simulink model "slvnvdemo_fuelsys_doorsreq"  (Simulink 7.6)
settings: Solver=ode45  SolverMode=SingleTasking  StartTime=0.0  StopTime=20  FixedStep=0.001  RelTol=1e-5  AbsTol=1e-6
model workspace (MAT data in the model file):
  A1 = [1 -0.740818220682]
  A2 = [1 -0.740818220682]
  A3 = [1 0 0 0]
  B1 = [8.76963147833 -8.51044969901]
  B2 = [0 0.259181779318]
  B3 = [1 0 0 0]
  DISABLED = 3
  hys = 25
  Ki = 0.012
  LOW = 1
  max_ego = 1.2
  max_press = 1
  max_speed = 628
  max_throt = 90
  min_press = 0.001
  min_throt = 3
  o2_t_thresh = 4.8
  press = [0.05 0.1 0.15 0.2 0.25 0.3 0.35 0.4 0.45 0.5 0.55 0.6 0.65 0.7 0.75 0.8 0.85 0.9 0.95]
  PressEst = [0.806253176324 0.553142316929 0.37151500209 0.277667903103 0.220198954207 0.181288665766 0.153200000489 0.115431020872 0.0913067476324 0.0746519188607 0.0625231108324 0.0533383634277 ... (306 elements, 18x17)]
  pumpCon = [-0.0556348 -0.0022828 0.0256932 0.0435188 0.0562692 0.0661194857143 0.0741572 0.08697 0.0972452 0.106070342857 0.1139892 0.121303866667 ... (342 elements, 18x19)]
  RICH = 2
  SpeedEst = [471.837839721 550.80940091 777.559313277 1080.9243499 1418.36795322 1769.7468768 2125.37309264 2480.20345067 2831.37796793 3177.14006959 3516.32917143 4064.90417867 ... (323 elements, 17x19)]
  SpeedVect = [50 75 100 125 150 175 200 250 300 350 400 450 500 600 700 800 900 1000]
  ThrotEst = [0 0 0 0 0 0 0 0 0 0 0 0 ... (342 elements, 18x19)]
  ThrotVect = [0 3 6 9 12 15 18 21 24 27 30 35 46 57 68 79 90]
  xzero = [0.0684931506849; 0.1; 0; 0]
  zero_thresh : num (value not decoded)
undefined symbols (not defined in the file or in its folder): DiscIntNeverNeededParam, sigbuilder_block
libraries: simulink x4, simulink_extras x3
Description:
  | This is a model of a fuel control system where Stateflow(R) is used to handle the fault management of the system.  The system modeled here contains four separate sensors: a throttle sensor, a speed sensor, an oxygen sensor, and a pressure sensor.  Each of these sensors is represented by a parallel state in Stateflow.  Each parallel state contains two substates, a normal state and a failed state (the exception being the oxygen sensor, which also contains a warmup state).
  | 
  | If any of the sensor readings is outside an acceptable range, then a fault is registered in Stateflow, and the substate of the corresponding subsystem transitions to the failed state.  If a subsystem recovers, it can transition back to the normal state.  The number of failures in the system at any given time is represented in the Sens_Failure_Counter parallel state.
  | 
  | The last parallel state in the Stateflow chart is called Fueling_Mode.  This state regulates the oxygen to fuel mixture ratio.  If a failure is detected, then the oxygen to fuel ratio is increased.  If multiple failures are detected, then the fuel system is disabled until there are no longer multiple failures in the system.
settings Model: RequirementInfo={'doors' '00001143' '1' 'false' 'DOORS Surrogate Item' '' ; 'other' 'fuelsys_req_docs\slvnvdemo_FuelSys_DesignDescription.docx' '' 'true' 'Design Description Microsoft Word Document' '' } %GIDa_b9f5e970_9947_4c5b_8209_982c9caa298e  reqMgrSettings="100 S'doors','misc'{{S'surrogatepath','savemodel','savesurrogate','updateLinks','doorsLinks2sl','slLinks2Doors','purgeDoors','purgeSimulink','detaillevel','surrogateId','synctime'{{T\"/DemoRMI/slvnvdemo_fuelsys_doorsreq\",M[0],M[0],M[0],M[0],M[0],M[0],M[0],M[6],T\"00001143\",T\"\"}},S'mode','pathStorage'{{T\"generic\",T\"modelRelative\"}}}}"  Creator=The MathWorks Inc.  CovMetricSettings=dcmtr  ExtModeTrigMode=oneshot  ExtModeArmWhenConnect=off  ExtModeAutoUpdateStatusClock=off
settings SolverCC: InsertRTBMode=Auto
settings DataIOCC: LimitDataPoints=off  SaveOutput=off  SaveTime=off
settings OptimizationCC: InlineInvariantSignals=on  InitFltsAndDblsToZero=on  EfficientMapNaN2IntZero=off
settings DebuggingCC: SaveWithParameterizedLinksMsg=none  SignalResolutionControl=TryResolveAllWithWarning  SolverPrmCheckMsg=none  MultiTaskDSMMsg=warning  MultiTaskCondExecSysMsg=none  IntegerOverflowMsg=none  StrictBusMsg=None
settings HardwareCC: TargetUnknown=on
settings SFSimCC: SimParseCustomCode=off
settings RTWCC: IncludeERTFirstTime=on
settings GRTTargetCC: TargetFcnLib=ansi_tfl_tmw.mat

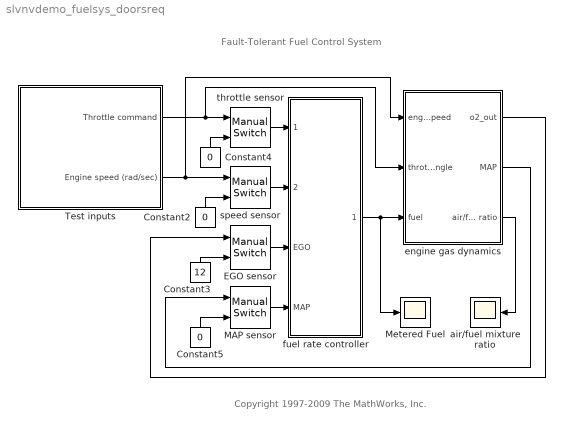
== system slvnvdemo_fuelsys_doorsreq ==
  note: Fault-Tolerant Fuel Control System
  note: Copyright 1997-2009 The MathWorks, Inc.
  Constant2 : Constant  RequirementInfo={'doors' '00001143' '2' 'false' 'DOORS Surrogate Item' '' } %GIDa_6f510076_839c_4984_a068_82184ea5f27a  Value=0
  Constant3 : Constant  RequirementInfo={'doors' '00001143' '3' 'false' 'DOORS Surrogate Item' '' } %GIDa_4aea0302_c695_4d64_8fee_9965b0b11529  Value=12
  Constant4 : Constant  RequirementInfo={'doors' '00001143' '4' 'false' 'DOORS Surrogate Item' '' } %GIDa_f16c33ef_29fe_45bd_a15f_c77a44a505fb  Value=0
  Constant5 : Constant  RequirementInfo={'doors' '00001143' '5' 'false' 'DOORS Surrogate Item' '' } %GIDa_53ad70e6_a414_4a38_8170_e2a41f36da5c  Value=0
  EGO sensor : simulink/Signal Routing/Manual Switch  RequirementInfo={'doors' '00001143' '6' 'false' 'DOORS Surrogate Item' '' } %GIDa_fc1de3a5_f710_44ee_8aab_8ba6d02ce341  SystemSampleTime=-1  sw=1  action=0  varsize=off
  MAP sensor : simulink/Signal Routing/Manual Switch  RequirementInfo={'doors' '00001143' '7' 'false' 'DOORS Surrogate Item' '' } %GIDa_9fc2c968_6068_49c6_968d_b08e363248b9  SystemSampleTime=-1  sw=1  action=0  varsize=off
  Metered Fuel : Scope
      settings: RequirementInfo={'doors' '00001143' '8' 'false' 'DOORS Surrogate Item' '' } %GIDa_681a171d_a3c5_4885_b64c_8848497df52d  TickLabels=on  TimeRange=20  YMin=0.75  YMax=2.25  DataFormat=Array
  Test inputs : Subsystem  Tag=STV Subsys  RequirementInfo={'doors' '00001143' '9' 'false' 'DOORS Surrogate Item' '' ; 'doors' '00001143' '10' 'false' 'DOORS Surrogate Item' '' } %GIDa_edea01b3_1c6d_4155_a72f_5a035e20164d  LoadFcn=sigbuilder_block('load');  StartFcn=sigbuilder_block('start');  StopFcn=sigbuilder_block('stop');  ClipboardFcn=sigbuilder_block('clipboard');  mask(Sigbuilder block){}
      mask help: Create and generate interchangeable groups of signals whose waveforms are piecewise linear.
      mask init:
      | if ~strcmp(get_param(bdroot(gcbh),'SimulationStatus'),'stopped') tuvar = sigbuilder_block('maskInit'); end
      settings: CopyFcn=sigbuilder_block('copy');  DeleteFcn=sigbuilder_block('delete');  ModelCloseFcn=sigbuilder_block('modelClose');  PreSaveFcn=sigbuilder_block('preSave');  NameChangeFcn=sigbuilder_block('namechange');  OpenFcn=sigbuilder_block('open',[764.25 127.5 550.5 399.75 ]);  CloseFcn=sigbuilder_block('close');
      mask Display: plot(0,0,100,100,[10,10,40,40,10],[80,20,20,80,80],[40,10],[50,50], [40,27,10],[65,72,56],[40,25,25,10],[28,28,43,43]);
  air/fuel mixture ratio : Scope
      settings: RequirementInfo={'doors' '00001143' '11' 'false' 'DOORS Surrogate Item' '' } %GIDa_eb27b04a_0dbf_4cdf_926f_da0d02353e65  TickLabels=on  TimeRange=20  YMin=11  YMax=16  DataFormat=Array
  engine gas dynamics : Subsystem  RequirementInfo={'doors' '00001143' '12' 'false' 'DOORS Surrogate Item' '' } %GIDa_1a392509_8e3f_4212_812a_096eaacb0e7b
  fuel rate controller : Subsystem  RequirementInfo={'doors' '00001143' '61' 'false' 'DOORS Surrogate Item' '' } %GIDa_1c1b78ad_f226_4b22_a092_d4af30d7278c
  speed sensor : simulink/Signal Routing/Manual Switch  RequirementInfo={'doors' '00001143' '234' 'false' 'DOORS Surrogate Item' '' } %GIDa_db4c3198_d72b_4db1_84d1_60b53fad8198  SystemSampleTime=-1  sw=1  action=0  varsize=off
  throttle sensor : simulink/Signal Routing/Manual Switch  RequirementInfo={'doors' '00001143' '235' 'false' 'DOORS Surrogate Item' '' } %GIDa_38ef20e4_d6ae_4cd9_b31a_0da7b200996a  SystemSampleTime=-1  sw=1  action=0  varsize=off
  wires:
  engine gas dynamics/3(air/fuel ratio) -> air/fuel mixture ratio/1
  Test inputs/2(Engine speed (rad/sec)) -> engine gas dynamics/1(engine speed), speed sensor/1
  MAP sensor/1 -> fuel rate controller/4(MAP)
  EGO sensor/1 -> fuel rate controller/3(EGO)
  speed sensor/1 -> fuel rate controller/2(engine speed)
  throttle sensor/1 -> fuel rate controller/1(throttle)
  fuel rate controller/1(fuel rate) -> engine gas dynamics/3(fuel), Metered Fuel/1
  engine gas dynamics/1(o2_out) -> EGO sensor/1
  Constant5/1 -> MAP sensor/2
  Constant3/1 -> EGO sensor/2
  Test inputs/1(Throttle command) -> engine gas dynamics/2(throttle angle), throttle sensor/1
  Constant2/1 -> speed sensor/2
  Constant4/1 -> throttle sensor/2
  engine gas dynamics/2(MAP) -> MAP sensor/1

== system slvnvdemo_fuelsys_doorsreq/Test inputs ==
  Demux : Demux  Tag=STV Demux  Outputs=2
  FromWs : FromWorkspace  Tag=STV FromWs  VariableName=tuvar  SampleTime=0  SigBuilderData=DataTag1  VnvData=DataTag2
      SigBuilderData=|
      | common.afterFinalStr = 'Extrapolate'
      | common.sampleTime = 0
      | dataSet(1).timeRange = [0 20]
      | dataSet(1).name = 'Normal operation'
      | dataSet(2).timeRange = [0 20]
      | dataSet(2).name = 'RPM sensor failure'
      | sbobj.Groups(1).Name = 'Normal operation'
      | sbobj.Groups(1).Signals(1).Name = 'Throttle command'
      | sbobj.Groups(1).Signals(1).XData = [0 0.5 1 1.5 2 2.5 3 3.5 4 4.5 5 5.5 6 6.5 7 7.5 8 8.5 9 9.5 10 10.5 11 11.5 12 12.5 13 13.5 14 14.5 15 15.5 16 16.5 17 17.5 18 18.5 19 19.5 20]
      | sbobj.Groups(1).Signals(1).YData = [15 18.5355339059 20 18.5355339059 15 11.4644660941 10 11.4644660941 15 18.5355339059 20 18.5355339059 15 11.4644660941 10 11.4644660941 15 18.5355339059 20 18.5355339059 15 11.4644660941 10 11.4644660941 15 18.5355339059 20 18.5355339059 15 11.4644660941 10 11.4644660941 15 18.5355339059 20 18.5355339059 15 11.4644660941 10 11.4644660941 15]
      | sbobj.Groups(1).Signals(2).Name = 'Engine speed (rad/sec)'
      | sbobj.Groups(1).Signals(2).XData = [0 20]
      | sbobj.Groups(1).Signals(2).YData = [300 300]
      | sbobj.Groups(2).Name = 'RPM sensor failure'
      | sbobj.Groups(2).Signals(1).Name = 'Throttle command'
      | sbobj.Groups(2).Signals(1).XData = [0 0.5 1 1.5 2 2.5 3 3.5 4 4.5 5 5.5 6 6.5 7 7.5 8 8.5 9 9.5 10 10.5 11 11.5 12 12.5 13 13.5 14 14.5 15 15.5 16 16.5 17 17.5 18 18.5 19 19.5 20]
      | sbobj.Groups(2).Signals(1).YData = [15 18.5355339059 20 18.5355339059 15 11.4644660941 10 11.4644660941 15 18.5355339059 20 18.5355339059 15 11.4644660941 10 11.4644660941 15 18.5355339059 20 18.5355339059 15 11.4644660941 10 11.4644660941 15 18.5355339059 20 18.5355339059 15 11.4644660941 10 11.4644660941 15 18.5355339059 20 18.5355339059 15 11.4644660941 10 11.4644660941 15]
      | sbobj.Groups(2).Signals(2).Name = 'Engine speed (rad/sec)'
      | sbobj.Groups(2).Signals(2).XData = [0 10 10 14 14 20]
      | sbobj.Groups(2).Signals(2).YData = [300 300 700 700 300 300]
  Throttle command : Outport  Tag=STV Outport
  Engine speed (rad/sec) : Outport  Tag=STV Outport  Port=2
  wires:
  Demux/1 -> Throttle command/1
  FromWs/1 -> Demux/1
  Demux/2 -> Engine speed (rad/sec)/1

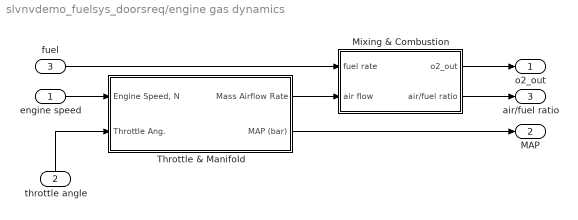
== system slvnvdemo_fuelsys_doorsreq/engine gas dynamics ==
  engine speed : Inport  RequirementInfo={'doors' '00001143' '13' 'false' 'DOORS Surrogate Item' '' } %GIDa_af43e267_eca7_4317_9a9e_118e96c8df3a
  throttle angle : Inport  RequirementInfo={'doors' '00001143' '14' 'false' 'DOORS Surrogate Item' '' } %GIDa_e17f4ea5_0288_401d_90f7_37f91cb17cef  Port=2
  fuel : Inport  RequirementInfo={'doors' '00001143' '15' 'false' 'DOORS Surrogate Item' '' } %GIDa_51f9453d_90e5_4716_8a70_66d58a29b78f  Port=3
  Mixing & Combustion : Subsystem  RequirementInfo={'doors' '00001143' '16' 'false' 'DOORS Surrogate Item' '' } %GIDa_b39f573e_5037_443c_be2b_1a4548c5c0e7
  Throttle & Manifold : Subsystem  RequirementInfo={'doors' '00001143' '26' 'false' 'DOORS Surrogate Item' '' } %GIDa_a2d66e4e_7a50_46f2_8e9d_462815b41651
  o2_out : Outport  RequirementInfo={'doors' '00001143' '58' 'false' 'DOORS Surrogate Item' '' } %GIDa_2b902bd2_437a_4448_b4ab_a1d7bbca09e4  InitialOutput=0
  MAP : Outport  RequirementInfo={'doors' '00001143' '59' 'false' 'DOORS Surrogate Item' '' } %GIDa_84abcf36_567c_4069_a0b2_4759d3edc095  Port=2  InitialOutput=0
  air/fuel ratio : Outport  RequirementInfo={'doors' '00001143' '60' 'false' 'DOORS Surrogate Item' '' } %GIDa_a523c5d4_fa31_4aa3_8903_8b83a3fe08ed  Port=3  InitialOutput=0
  wires:
  Throttle & Manifold/1(Mass Airflow Rate) -> Mixing & Combustion/2(air flow)
  fuel/1 -> Mixing & Combustion/1(fuel rate)
  engine speed/1 -> Throttle & Manifold/1("Engine Speed, N")
  throttle angle/1 -> Throttle & Manifold/2(Throttle Ang.)
  Mixing & Combustion/2(air/fuel ratio) -> air/fuel ratio/1
  Throttle & Manifold/2(MAP (bar)) -> MAP/1
  Mixing & Combustion/1(o2_out) -> o2_out/1

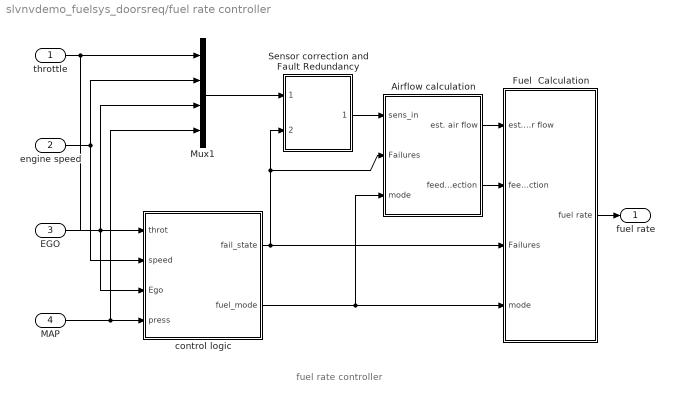
== system slvnvdemo_fuelsys_doorsreq/fuel rate controller ==
  note: fuel rate controller
  throttle : Inport  RequirementInfo="{'doors' '00001143' '62' 'false' 'DOORS Surrogate Item' '' ; 'linktype_rmi_doors' '00001140 (/DemoRMI/FuelSys Design Description)' '#24' 'true' '1.1.1.1  Throttle Sensor' 'design' } %GIDa_9cf99e51_43b0_47f7_8264_f2235da8c515"
  engine speed : Inport  RequirementInfo={'doors' '00001143' '63' 'false' 'DOORS Surrogate Item' '' } %GIDa_5b17eedf_e9cf_48a4_ac44_7982ccd64ca2  Port=2
  EGO : Inport  RequirementInfo={'doors' '00001143' '64' 'false' 'DOORS Surrogate Item' '' } %GIDa_6fef81ac_5f90_4a8e_828a_423a97d08b10  Port=3
  MAP : Inport  RequirementInfo="{'doors' '00001143' '65' 'false' 'DOORS Surrogate Item' '' ; 'linktype_rmi_doors' '00001140 (/DemoRMI/FuelSys Design Description)' '#28' 'true' '1.1.1.2  Manifold Absolute Pressure Sensor ' 'design' } %GIDa_4c5e0388_e181_4bd6_b11e_64e9ecd3fbd1"  Port=4
  Airflow calculation : Subsystem  RequirementInfo="{'doors' '00001143' '66' 'false' 'DOORS Surrogate Item' '' ; 'linktype_rmi_doors' '00001140 (/DemoRMI/FuelSys Design Description)' '#47' 'true' '1.2.1  Mass airflow estimation ' 'design' } %GIDa_e5d50a88_c804_4174_8af1_23d9a3e696a6"
  Fuel  Calculation : Subsystem  RequirementInfo={'doors' '00001143' '92' 'false' 'DOORS Surrogate Item' '' } %GIDa_34097df7_79d7_4c80_bbb4_c8c21d1d631f
  Mux1 : Mux  RequirementInfo={'doors' '00001143' '134' 'false' 'DOORS Surrogate Item' '' } %GIDa_83488a2d_fa56_4d28_96fb_fd2056fe6956
  Sensor correction and Fault Redundancy : Subsystem  RequirementInfo={'doors' '00001143' '135' 'false' 'DOORS Surrogate Item' '' } %GIDa_518d74c7_343f_4c0b_a3e5_2212a7618a1e
  control logic : Stateflow chart  Description=Stateflow diagram to determine control system operating mode  RequirementInfo={'doors' '00001143' '168' 'false' 'DOORS Surrogate Item' '' } %GIDa_5c71245a_39cc_4b2d_a7dc_93f0d532609e  TreatAsAtomicUnit=on
  fuel rate : Outport  RequirementInfo={'doors' '00001143' '233' 'false' 'DOORS Surrogate Item' '' } %GIDa_b9667016_fb09_447c_b6a0_1390dfc20aea  InitialOutput=0
  wires:
  MAP/1 -> Mux1/4, control logic/4(press)
  EGO/1 -> Mux1/3, control logic/3(Ego)
  engine speed/1 -> Mux1/2, control logic/2(speed)
  throttle/1 -> Mux1/1, control logic/1(throt)
  Mux1/1 -> Sensor correction and Fault Redundancy/1(Sensors)
  control logic/2(fuel_mode) -> Fuel  Calculation/4(mode), Airflow calculation/3(mode)
  Airflow calculation/2(feedback correction) -> Fuel  Calculation/2(feedback correction)
  Fuel  Calculation/1(fuel rate) -> fuel rate/1
  Airflow calculation/1(est. air flow) -> Fuel  Calculation/1(est. air flow)
  Sensor correction and Fault Redundancy/1(Corrected) -> Airflow calculation/1(sens_in)
  control logic/1(fail_state) -> Sensor correction and Fault Redundancy/2(Failures), Airflow calculation/2(Failures), Fuel  Calculation/3(Failures)

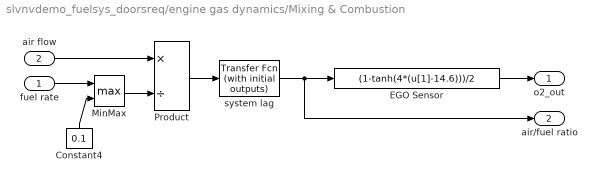
== system slvnvdemo_fuelsys_doorsreq/engine gas dynamics/Mixing & Combustion ==
  fuel rate : Inport  RequirementInfo={'doors' '00001143' '17' 'false' 'DOORS Surrogate Item' '' } %GIDa_a0da4f9a_920a_433c_bc96_8906b222f2c5
  air flow : Inport  RequirementInfo={'doors' '00001143' '18' 'false' 'DOORS Surrogate Item' '' } %GIDa_5caa34b4_a16f_4465_a750_f963464c11ad  Port=2
  Constant4 : Constant  RequirementInfo={'doors' '00001143' '19' 'false' 'DOORS Surrogate Item' '' } %GIDa_2bd17625_1ccb_44ba_a95c_a9230dfb67c2  Value=0.1
  EGO Sensor : Fcn  RequirementInfo={'doors' '00001143' '20' 'false' 'DOORS Surrogate Item' '' } %GIDa_6af401bd_9892_45e5_a1d1_0ec7c7cf995e  Expr=(1-tanh(4*(u[1]-14.6)))/2
  MinMax : MinMax  RequirementInfo={'doors' '00001143' '21' 'false' 'DOORS Surrogate Item' '' } %GIDa_6d9700e5_4410_4a4b_83fd_395721c529a2  Function=max  Inputs=2  SaturateOnIntegerOverflow=on  InputSameDT=on
  Product : Product  RequirementInfo={'doors' '00001143' '22' 'false' 'DOORS Surrogate Item' '' } %GIDa_088236aa_e2e4_4ea4_9127_1588bf7dce42  Inputs=*/  SaturateOnIntegerOverflow=on  RndMeth=Zero  InputSameDT=on  OutDataTypeStr=Inherit: Same as first input
  system lag : simulink_extras/Additional Linear/Transfer Fcn (with initial outputs)  RequirementInfo={'doors' '00001143' '23' 'false' 'DOORS Surrogate Item' '' } %GIDa_4fc8d989_be95_4469_a582_179e8d71f6fb  SystemSampleTime=-1  N=3  D=[1 3]  Y0=1/14.6  U0=1/14.6
  o2_out : Outport  RequirementInfo={'doors' '00001143' '24' 'false' 'DOORS Surrogate Item' '' } %GIDa_db90f587_e1ae_4b5c_a93b_c6026d9cd193  InitialOutput=0
  air/fuel ratio : Outport  RequirementInfo={'doors' '00001143' '25' 'false' 'DOORS Surrogate Item' '' } %GIDa_ccc3460d_06a5_47de_9c88_91db6cd6257a  Port=2  InitialOutput=0
  wires:
  Constant4/1 -> MinMax/2
  fuel rate/1 -> MinMax/1
  MinMax/1 -> Product/2
  Product/1 -> system lag/1
  system lag/1 -> air/fuel ratio/1, EGO Sensor/1
  EGO Sensor/1 -> o2_out/1
  air flow/1 -> Product/1

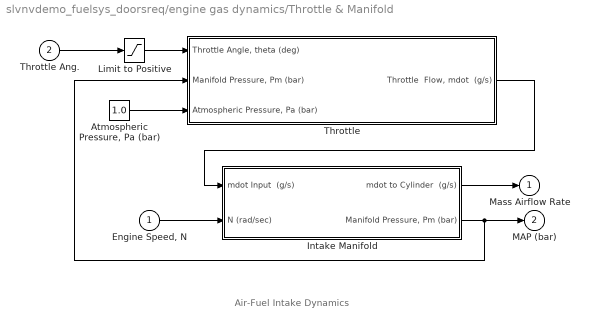
== system slvnvdemo_fuelsys_doorsreq/engine gas dynamics/Throttle & Manifold ==
  note: Air-Fuel Intake Dynamics
  "Engine Speed, N" : Inport  RequirementInfo={'doors' '00001143' '27' 'false' 'DOORS Surrogate Item' '' } %GIDa_5ade23e6_58b2_41f7_a122_1e2e0c1b17b3
  Throttle Ang. : Inport  RequirementInfo={'doors' '00001143' '28' 'false' 'DOORS Surrogate Item' '' } %GIDa_2144ca48_684d_4403_a2ab_d151350c3292  Port=2
  "Atmospheric Pressure, Pa (bar)" : Constant  RequirementInfo={'doors' '00001143' '29' 'false' 'DOORS Surrogate Item' '' } %GIDa_1a9422a6_df72_468a_8215_e86ed5f6b7c8  Value=1.0
  Intake Manifold : Subsystem  RequirementInfo={'doors' '00001143' '30' 'false' 'DOORS Surrogate Item' '' } %GIDa_30547359_4c19_480c_b03f_94e0e8057713
  Limit to Positive : Saturate  RequirementInfo={'doors' '00001143' '40' 'false' 'DOORS Surrogate Item' '' } %GIDa_d18fb706_3f5b_4d8c_a6ba_6d66caf2459d  UpperLimit=inf  LowerLimit=0
  Throttle : Subsystem  RequirementInfo={'doors' '00001143' '41' 'false' 'DOORS Surrogate Item' '' } %GIDa_6d2f1b09_850e_498a_ba3e_b75a873ac8b1
  Mass Airflow Rate : Outport  RequirementInfo={'doors' '00001143' '56' 'false' 'DOORS Surrogate Item' '' } %GIDa_bfc60757_b652_41dd_9950_22ed52e7ad5a  InitialOutput=0
  MAP (bar) : Outport  RequirementInfo={'doors' '00001143' '57' 'false' 'DOORS Surrogate Item' '' } %GIDa_005c3ac9_21df_4f04_a20c_8b9399e94d45  Port=2  InitialOutput=0
  wires:
  Limit to Positive/1 -> Throttle/1("Throttle Angle, theta (deg)")
  Throttle Ang./1 -> Limit to Positive/1
  Throttle/1("Throttle  Flow, mdot  (g/s)") -> Intake Manifold/1(mdot Input  (g/s))
  "Engine Speed, N"/1 -> Intake Manifold/2(N (rad/sec))
  Intake Manifold/1(mdot to Cylinder  (g/s)) -> Mass Airflow Rate/1
  "Atmospheric Pressure, Pa (bar)"/1 -> Throttle/3("Atmospheric Pressure, Pa (bar) ")
  Intake Manifold/2("Manifold Pressure, Pm (bar)") -> Throttle/2("Manifold Pressure, Pm (bar)"), MAP (bar)/1

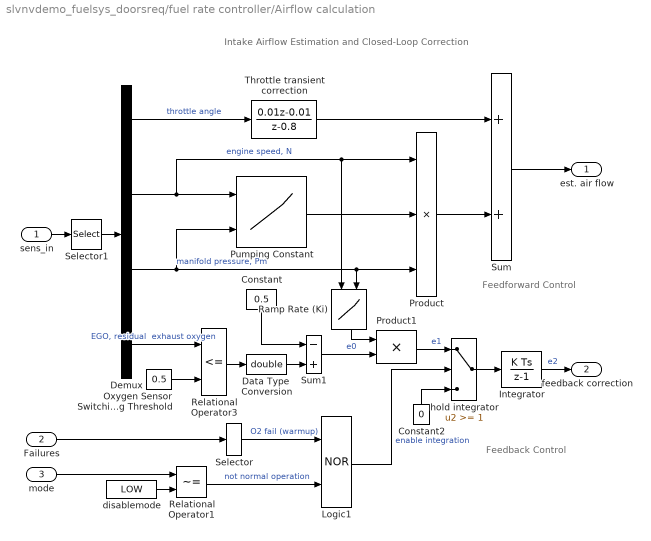
== system slvnvdemo_fuelsys_doorsreq/fuel rate controller/Airflow calculation ==
  note: Intake Airflow Estimation and Closed-Loop Correction
  note: Feedback Control
  note: Feedforward Control
  sens_in : Inport  RequirementInfo={'doors' '00001143' '67' 'false' 'DOORS Surrogate Item' '' } %GIDa_89c385b5_6d02_4edb_b95d_519ab4f6fcae
  Failures : Inport  RequirementInfo={'doors' '00001143' '68' 'false' 'DOORS Surrogate Item' '' } %GIDa_ba8b6ad3_a9c1_47be_b489_b5d91562cb0f  Port=2
  mode : Inport  RequirementInfo={'doors' '00001143' '69' 'false' 'DOORS Surrogate Item' '' } %GIDa_3d500005_c122_401a_8ca5_74c094964693  Port=3
  Constant : Constant  RequirementInfo={'doors' '00001143' '70' 'false' 'DOORS Surrogate Item' '' } %GIDa_513be1e0_2f3c_4ead_8fb6_4a7e5e8d18c8  Value=0.5
  Constant2 : Constant  RequirementInfo={'doors' '00001143' '71' 'false' 'DOORS Surrogate Item' '' } %GIDa_240682be_d736_4821_ab41_6fff13a8902b  Value=0
  Data Type  Conversion : DataTypeConversion  RequirementInfo={'doors' '00001143' '72' 'false' 'DOORS Surrogate Item' '' } %GIDa_ba098232_e5b8_40af_b3fd_9d8329a5a882  OutDataTypeStr=double  SaturateOnIntegerOverflow=on  RndMeth=Zero
  Demux : Demux  RequirementInfo={'doors' '00001143' '73' 'false' 'DOORS Surrogate Item' '' } %GIDa_f63eecf9_e4ef_42a6_8242_bd70091fe0ba
  Integrator : DiscreteIntegrator  RequirementInfo={'doors' '00001143' '74' 'false' 'DOORS Surrogate Item' '' } %GIDa_05798af3_2708_4e0e_a823_98ae6a074864  InitialCondition=-0.01  SampleTime=.01  ICPrevOutput=DiscIntNeverNeededParam  ICPrevScaledInput=DiscIntNeverNeededParam
  Logic1 : Logic  RequirementInfo={'doors' '00001143' '75' 'false' 'DOORS Surrogate Item' '' } %GIDa_7b2f8e35_d023_46b0_84cb_e56d63e4987f  Operator=NOR
  Oxygen Sensor Switching Threshold : Constant  RequirementInfo={'doors' '00001143' '76' 'false' 'DOORS Surrogate Item' '' } %GIDa_e9473781_d856_49c2_a2f4_26f4486be72c  Value=0.5
  Product : Product  RequirementInfo={'doors' '00001143' '77' 'false' 'DOORS Surrogate Item' '' } %GIDa_c2220dad_1bb2_47d5_a345_19450686b761  Inputs=3  SaturateOnIntegerOverflow=on  RndMeth=Zero  InputSameDT=on  OutDataTypeStr=Inherit: Same as first input
  Product1 : Product  RequirementInfo={'doors' '00001143' '78' 'false' 'DOORS Surrogate Item' '' } %GIDa_4a0efd8c_4cf9_496f_b7ee_0e2e7d4d336c  SaturateOnIntegerOverflow=on  RndMeth=Zero  InputSameDT=on  OutDataTypeStr=Inherit: Same as first input
  Pumping Constant : Lookup2D  RequirementInfo={'doors' '00001143' '79' 'false' 'DOORS Surrogate Item' '' } %GIDa_83ce71ba_24f4_4658_a901_8e8800a19d30  RowIndex=SpeedVect  ColumnIndex=press  Table=pumpCon  SaturateOnIntegerOverflow=on  InputSameDT=on
  Ramp Rate (Ki) : Lookup2D  RequirementInfo={'doors' '00001143' '80' 'false' 'DOORS Surrogate Item' '' } %GIDa_6d7274a7_0fcb_4051_80d3_51bd87243910  RowIndex=[100:100:500]  ColumnIndex=[0:0.2:1]  Table=[1:5]'*[1:6]*Ki  SaturateOnIntegerOverflow=on  InputSameDT=on
  Relational Operator1 : RelationalOperator  RequirementInfo={'doors' '00001143' '81' 'false' 'DOORS Surrogate Item' '' } %GIDa_d42f50d1_b9f3_459d_9348_e65432ae7b35  Operator=~=  InputSameDT=on
  Relational Operator3 : RelationalOperator  RequirementInfo={'doors' '00001143' '82' 'false' 'DOORS Surrogate Item' '' ; 'other' 'fuelsys_req_docs\slvnvdemo_FuelSys_RequirementsSpecification.docx' '@Simulink_requirement_item_4' 'true' 'High Oxygen Level' 'word' } %GIDa_1ac98a75_43e6_4298_867c_a36938fb0ef3  Operator=<=  InputSameDT=on
  Selector : Selector  RequirementInfo={'doors' '00001143' '83' 'false' 'DOORS Surrogate Item' '' } %GIDa_e8a7ff9d_8131_4a85_ac0e_07023a5602a3  InputPortWidth=4  IndexOptions=Index vector (dialog)  Indices=3  OutputSizes=1
  Selector1 : Selector  RequirementInfo={'doors' '00001143' '84' 'false' 'DOORS Surrogate Item' '' } %GIDa_93a9e621_e801_42f1_981c_585598a06b87  InputPortWidth=4  IndexOptions=Index vector (dialog)  Indices=[1 2 4 3]  OutputSizes=1
  Sum : Sum  RequirementInfo={'doors' '00001143' '85' 'false' 'DOORS Surrogate Item' '' } %GIDa_0cb313c7_e7b5_4516_9821_4a35e7126f23  Inputs=2  SaturateOnIntegerOverflow=on  InputSameDT=on  OutDataTypeStr=Inherit: Same as first input
  Sum1 : Sum  RequirementInfo={'doors' '00001143' '86' 'false' 'DOORS Surrogate Item' '' } %GIDa_ad1102f7_93b4_4b35_9511_d9762f06c4cb  Inputs=-+  SaturateOnIntegerOverflow=on  InputSameDT=on  OutDataTypeStr=Inherit: Same as first input
  Throttle transient correction : DiscreteTransferFcn  RequirementInfo={'doors' '00001143' '87' 'false' 'DOORS Surrogate Item' '' } %GIDa_87026890_b4cc_41c3_b0fc_686b49967b3d  Numerator=[0.01 -0.01]  Denominator=[1 -0.8]  SampleTime=.01
  disablemode : Constant  RequirementInfo={'doors' '00001143' '88' 'false' 'DOORS Surrogate Item' '' } %GIDa_d1a818ea_d888_4109_8d00_13968bc5a7b4  Value=LOW
  hold integrator : Switch  RequirementInfo={'doors' '00001143' '89' 'false' 'DOORS Surrogate Item' '' } %GIDa_411a4247_0314_4751_b6a6_ba3abd6a85d2  Threshold=1  SaturateOnIntegerOverflow=on  InputSameDT=on
  est. air flow : Outport  RequirementInfo={'doors' '00001143' '90' 'false' 'DOORS Surrogate Item' '' } %GIDa_beee977a_9fb2_49c8_9ccb_2733353ee4da  InitialOutput=0
  feedback correction : Outport  RequirementInfo={'doors' '00001143' '91' 'false' 'DOORS Surrogate Item' '' ; 'other' 'fuelsys_req_docs\slvnvdemo_FuelSys_RequirementsSpecification.docx' '@Simulink_requirement_item_5' 'true' 'Fuel-rich Mixture' 'word' } %GIDa_28432839_4df5_49d8_a247_1a6d4bca56be  Port=2  InitialOutput=0
  wires:
  Integrator/1 -> feedback correction/1  "e2"
  mode/1 -> Relational Operator1/1
  sens_in/1 -> Selector1/1
  Pumping Constant/1 -> Product/2
  Product/1 -> Sum/2
  Demux/3 -> Ramp Rate (Ki)/2, Product/3, Pumping Constant/2  "manifold pressure, Pm"
  Demux/2 -> Pumping Constant/1, Product/1, Ramp Rate (Ki)/1  "engine speed, N"
  Selector1/1 -> Demux/1
  Throttle transient correction/1 -> Sum/1
  Sum/1 -> est. air flow/1
  Demux/1 -> Throttle transient correction/1  "throttle angle"
  Selector/1 -> Logic1/1  "O2 fail (warmup)"
  Failures/1 -> Selector/1
  disablemode/1 -> Relational Operator1/2
  Relational Operator1/1 -> Logic1/2  "not normal operation"
  Demux/4 -> Relational Operator3/1  "EGO, residual  exhaust oxygen"
  Oxygen Sensor Switching Threshold/1 -> Relational Operator3/2
  Constant/1 -> Sum1/1
  Ramp Rate (Ki)/1 -> Product1/1
  Constant2/1 -> hold integrator/3
  Product1/1 -> hold integrator/1  "e1"
  hold integrator/1 -> Integrator/1
  Logic1/1 -> hold integrator/2  "enable integration"
  Sum1/1 -> Product1/2  "e0"
  Relational Operator3/1 -> Data Type  Conversion/1
  Data Type  Conversion/1 -> Sum1/2

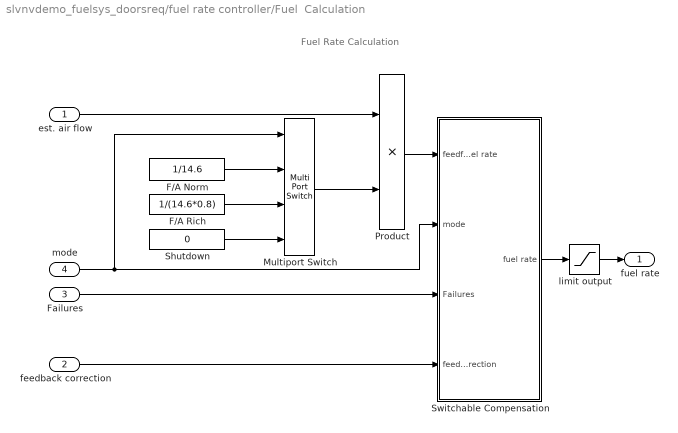
== system slvnvdemo_fuelsys_doorsreq/fuel rate controller/Fuel  Calculation ==
  note: Fuel Rate Calculation
  est. air flow : Inport  RequirementInfo={'doors' '00001143' '93' 'false' 'DOORS Surrogate Item' '' } %GIDa_84c231cb_6fd2_4ab8_a034_7560db01e73c
  feedback correction : Inport  RequirementInfo={'doors' '00001143' '94' 'false' 'DOORS Surrogate Item' '' } %GIDa_d5fbd09e_7cb8_42e1_923f_746b761ee62c  Port=2
  Failures : Inport  RequirementInfo={'doors' '00001143' '95' 'false' 'DOORS Surrogate Item' '' } %GIDa_55f44856_7460_492a_814a_a18b491dc4a0  Port=3
  mode : Inport  RequirementInfo={'doors' '00001143' '96' 'false' 'DOORS Surrogate Item' '' } %GIDa_3d971ec4_266e_49a8_9e91_dea383616b01  Port=4
  F/A Norm : Constant  RequirementInfo={'doors' '00001143' '97' 'false' 'DOORS Surrogate Item' '' } %GIDa_4a1a549c_eac8_4330_ac5b_48e08ff8e304  Value=1/14.6
  F/A Rich : Constant  RequirementInfo={'doors' '00001143' '98' 'false' 'DOORS Surrogate Item' '' } %GIDa_b6019cf7_42be_410a_8534_248d8790a64b  Value=1/(14.6*0.8)
  Multiport Switch : MultiPortSwitch  RequirementInfo={'doors' '00001143' '99' 'false' 'DOORS Surrogate Item' '' } %GIDa_11e58c93_2870_4797_aca4_4e150ec1c365  zeroidx=off  SaturateOnIntegerOverflow=on  InputSameDT=on
  Product : Product  RequirementInfo={'doors' '00001143' '100' 'false' 'DOORS Surrogate Item' '' } %GIDa_780ddfcf_d625_49de_8e61_f1cc814c276e  SaturateOnIntegerOverflow=on  RndMeth=Zero  InputSameDT=on  OutDataTypeStr=Inherit: Same as first input
  Shutdown : Constant  RequirementInfo={'doors' '00001143' '101' 'false' 'DOORS Surrogate Item' '' } %GIDa_f1fe4116_6399_41c2_8df8_a0ae40ab3b2d  Value=0
  Switchable Compensation : Subsystem  RequirementInfo={'doors' '00001143' '102' 'false' 'DOORS Surrogate Item' '' } %GIDa_6c1655bd_66cf_41ac_b937_2f19fc229125
  limit output : Saturate  RequirementInfo={'doors' '00001143' '132' 'false' 'DOORS Surrogate Item' '' } %GIDa_091a4f38_2142_44bb_987d_764ac9ca65e0  UpperLimit=100  LowerLimit=0
  fuel rate : Outport  RequirementInfo={'doors' '00001143' '133' 'false' 'DOORS Surrogate Item' '' } %GIDa_6fa91f2e_9b2e_47c8_800e_34e1f0ff4795  InitialOutput=0
  wires:
  limit output/1 -> fuel rate/1
  feedback correction/1 -> Switchable Compensation/4(feedback correction)
  Shutdown/1 -> Multiport Switch/4
  F/A Rich/1 -> Multiport Switch/3
  F/A Norm/1 -> Multiport Switch/2
  est. air flow/1 -> Product/1
  Multiport Switch/1 -> Product/2
  mode/1 -> Switchable Compensation/2(mode), Multiport Switch/1
  Failures/1 -> Switchable Compensation/3(Failures)
  Product/1 -> Switchable Compensation/1(feedforward fuel rate)
  Switchable Compensation/1(fuel rate) -> limit output/1

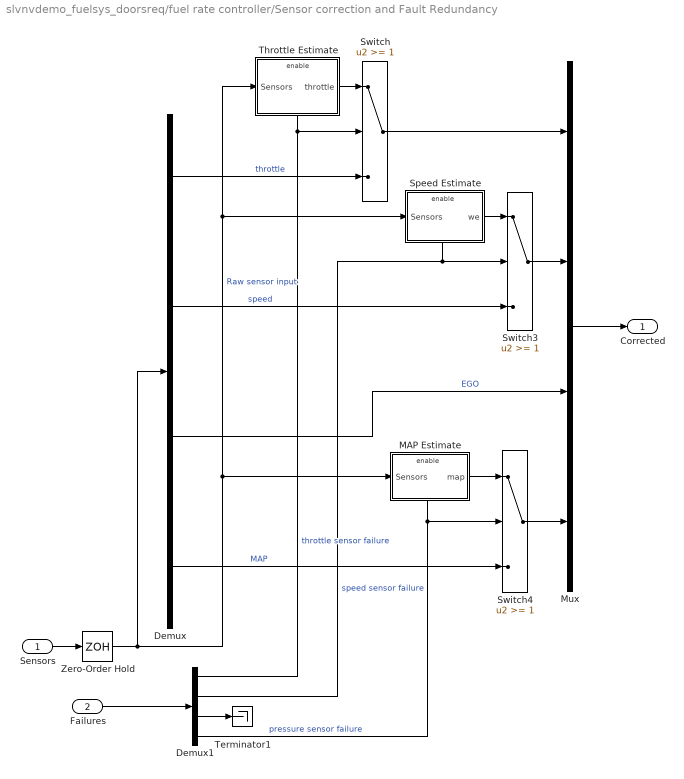
== system slvnvdemo_fuelsys_doorsreq/fuel rate controller/Sensor correction and Fault Redundancy ==
  Sensors : Inport  RequirementInfo={'doors' '00001143' '136' 'false' 'DOORS Surrogate Item' '' } %GIDa_836fb7ae_51c5_4078_bdf4_aa90711b96db
  Failures : Inport  RequirementInfo={'doors' '00001143' '137' 'false' 'DOORS Surrogate Item' '' } %GIDa_a7c57e9f_a424_4f44_897d_bfe0bb2db60c  Port=2
  Demux : Demux  RequirementInfo={'doors' '00001143' '138' 'false' 'DOORS Surrogate Item' '' } %GIDa_fc7d630c_81bb_4c1c_91ff_f1dab8db1463
  Demux1 : Demux  RequirementInfo={'doors' '00001143' '139' 'false' 'DOORS Surrogate Item' '' } %GIDa_39b82fb9_807c_47a8_9e19_36107efd9e75
  MAP Estimate : Subsystem  RequirementInfo="{'doors' '00001143' '140' 'false' 'DOORS Surrogate Item' '' ; 'linktype_rmi_doors' '00001140 (/DemoRMI/FuelSys Design Description)' '#69' 'true' '1.3.1.3  Manifold pressure failure mode ' 'design' } %GIDa_6fbafa07_e55c_40e6_b495_fca012362a9e"
  Mux : Mux  RequirementInfo={'doors' '00001143' '147' 'false' 'DOORS Surrogate Item' '' } %GIDa_c6c031c1_f49b_45b8_a1b4_e4d6c3da0abb
  Speed Estimate : Subsystem  RequirementInfo={'doors' '00001143' '148' 'false' 'DOORS Surrogate Item' '' } %GIDa_caec6c13_d6e7_456c_b0b6_2356949be5de
  Switch : Switch  RequirementInfo={'doors' '00001143' '155' 'false' 'DOORS Surrogate Item' '' } %GIDa_d63da140_e9cc_4c96_8c16_cb05db020237  Threshold=1  SaturateOnIntegerOverflow=on  InputSameDT=on
  Switch3 : Switch  RequirementInfo={'doors' '00001143' '156' 'false' 'DOORS Surrogate Item' '' } %GIDa_3faca5ab_a69e_4439_adea_53e03cfb7e28  Threshold=1  SaturateOnIntegerOverflow=on  InputSameDT=on
  Switch4 : Switch  RequirementInfo={'doors' '00001143' '157' 'false' 'DOORS Surrogate Item' '' } %GIDa_5983fa3f_f5fe_4476_a558_eebc3fbee84e  Threshold=1  SaturateOnIntegerOverflow=on  InputSameDT=on
  Terminator1 : Terminator
      settings: RequirementInfo="{'doors' '00001143' '158' 'false' 'DOORS Surrogate Item' '' ; 'linktype_rmi_doors' '00001140 (/DemoRMI/FuelSys Design Description)' '#84' 'true' '1.3.1.7   Fault Redundancy - section deleted' 'design' } %GIDa_4f68be0a_6cac_4fa2_8385_def99a25285d"
  Throttle Estimate : Subsystem  RequirementInfo={'doors' '00001143' '159' 'false' 'DOORS Surrogate Item' '' } %GIDa_ecbd61d6_16c6_4665_b9b7_fea316d2368c
  Zero-Order Hold : ZeroOrderHold  RequirementInfo={'doors' '00001143' '166' 'false' 'DOORS Surrogate Item' '' } %GIDa_61b624f9_99c0_42bd_bdd2_824012bc530f  SampleTime=0.01
  Corrected : Outport  RequirementInfo={'doors' '00001143' '167' 'false' 'DOORS Surrogate Item' '' } %GIDa_b1f488da_18db_40a4_8ef6_04b78afa74e8  InitialOutput=0
  wires:
  Sensors/1 -> Zero-Order Hold/1
  MAP Estimate/1(map) -> Switch4/1
  Demux/4 -> Switch4/3  "MAP"
  Switch4/1 -> Mux/4
  Demux1/4 -> Switch4/2, MAP Estimate/Enable  "pressure sensor failure"
  Demux1/2 -> Switch3/2, Speed Estimate/Enable  "speed sensor failure"
  Speed Estimate/1(we) -> Switch3/1
  Demux/2 -> Switch3/3  "speed"
  Switch3/1 -> Mux/2
  Demux1/1 -> Switch/2, Throttle Estimate/Enable  "throttle sensor failure"
  Demux1/3 -> Terminator1/1
  Throttle Estimate/1(throttle) -> Switch/1
  Demux/1 -> Switch/3  "throttle"
  Failures/1 -> Demux1/1
  Zero-Order Hold/1 -> Demux/1, Throttle Estimate/1(Sensors), Speed Estimate/1(Sensors), MAP Estimate/1(Sensors)  "Raw sensor input"
  Switch/1 -> Mux/1
  Demux/3 -> Mux/3  "EGO"
  Mux/1 -> Corrected/1

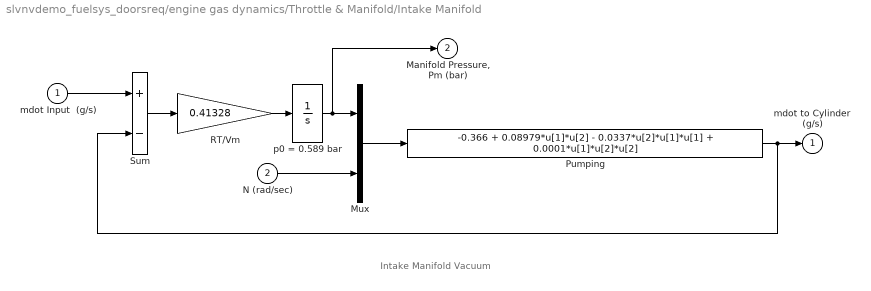
== system slvnvdemo_fuelsys_doorsreq/engine gas dynamics/Throttle & Manifold/Intake Manifold ==
  note: Intake Manifold Vacuum
  mdot Input  (g/s) : Inport  RequirementInfo={'doors' '00001143' '31' 'false' 'DOORS Surrogate Item' '' } %GIDa_37a540f9_db37_4391_9979_85eb33975dd4
  N (rad/sec) : Inport  RequirementInfo={'doors' '00001143' '32' 'false' 'DOORS Surrogate Item' '' } %GIDa_be8ac575_49e8_4364_8f01_88ac4ecdbfcb  Port=2
  Mux : Mux  RequirementInfo={'doors' '00001143' '33' 'false' 'DOORS Surrogate Item' '' } %GIDa_ced02565_f23d_415b_8b68_aad0a465d177  Inputs=2
  Pumping : Fcn  RequirementInfo={'doors' '00001143' '34' 'false' 'DOORS Surrogate Item' '' } %GIDa_d4034506_89aa_4b2b_a173_2ac65f42e42d  Expr=-0.366 + 0.08979*u[1]*u[2] - 0.0337*u[2]*u[1]*u[1] + 0.0001*u[1]*u[2]*u[2]
  RT/Vm : Gain  RequirementInfo={'doors' '00001143' '35' 'false' 'DOORS Surrogate Item' '' } %GIDa_7da24046_755d_4126_a054_0c2c208d5aa3  Gain=0.41328  SaturateOnIntegerOverflow=on  OutDataTypeStr=Inherit: Same as input  ParamDataTypeStr=Inherit: Same as input
  Sum : Sum  RequirementInfo={'doors' '00001143' '36' 'false' 'DOORS Surrogate Item' '' } %GIDa_48d11bc6_4799_47e1_8974_91e034a28f47  Inputs=+-  SaturateOnIntegerOverflow=on  InputSameDT=on  OutDataTypeStr=Inherit: Same as first input
  p0 = 0.589 bar : Integrator  RequirementInfo={'doors' '00001143' '37' 'false' 'DOORS Surrogate Item' '' } %GIDa_44f6ad13_1969_48a6_a02f_758c6d6fae4d  InitialCondition=.589
  mdot to Cylinder  (g/s) : Outport  RequirementInfo={'doors' '00001143' '38' 'false' 'DOORS Surrogate Item' '' } %GIDa_9a35e96f_7a5f_4a97_ba1f_57b2bb06e5ab  InitialOutput=0
  "Manifold Pressure, Pm (bar)" : Outport  RequirementInfo={'doors' '00001143' '39' 'false' 'DOORS Surrogate Item' '' } %GIDa_529e9053_2e73_4e92_96ac_24f4c0a3fdd7  Port=2  InitialOutput=0
  wires:
  mdot Input  (g/s)/1 -> Sum/1
  RT/Vm/1 -> p0 = 0.589 bar/1
  N (rad/sec)/1 -> Mux/2
  Mux/1 -> Pumping/1
  p0 = 0.589 bar/1 -> Mux/1, "Manifold Pressure, Pm (bar)"/1
  Sum/1 -> RT/Vm/1
  Pumping/1 -> Sum/2, mdot to Cylinder  (g/s)/1

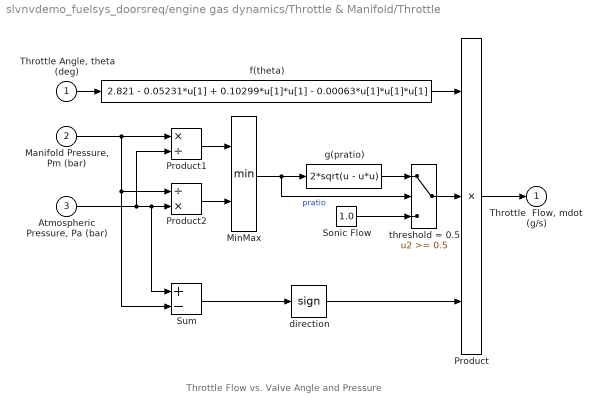
== system slvnvdemo_fuelsys_doorsreq/engine gas dynamics/Throttle & Manifold/Throttle ==
  note: Throttle Flow vs. Valve Angle and Pressure
  "Throttle Angle, theta (deg)" : Inport  RequirementInfo={'doors' '00001143' '42' 'false' 'DOORS Surrogate Item' '' } %GIDa_3217772c_31d4_4ae0_957e_f8c9c97ba270
  "Manifold Pressure, Pm (bar)" : Inport  RequirementInfo={'doors' '00001143' '43' 'false' 'DOORS Surrogate Item' '' } %GIDa_058de56f_1496_4156_a51b_c4dd1000c4d2  Port=2
  "Atmospheric Pressure, Pa (bar) " : Inport  RequirementInfo={'doors' '00001143' '44' 'false' 'DOORS Surrogate Item' '' } %GIDa_eb699b50_6c3f_4cc4_8db5_1aa3fc9bd274  Port=3
  MinMax : MinMax  RequirementInfo={'doors' '00001143' '45' 'false' 'DOORS Surrogate Item' '' } %GIDa_34e903c9_621a_4fc1_b827_3591070eab72  Inputs=2  SaturateOnIntegerOverflow=on  InputSameDT=on
  Product : Product  RequirementInfo={'doors' '00001143' '46' 'false' 'DOORS Surrogate Item' '' } %GIDa_a51026b6_3650_419c_9d43_cc4d448e98c6  Inputs=3  SaturateOnIntegerOverflow=on  RndMeth=Zero  InputSameDT=on  OutDataTypeStr=Inherit: Same as first input
  Product1 : Product  RequirementInfo={'doors' '00001143' '47' 'false' 'DOORS Surrogate Item' '' } %GIDa_a34e2897_b7c3_48be_9aa8_4c5af01e36ae  Inputs=*/  SaturateOnIntegerOverflow=on  RndMeth=Zero  InputSameDT=on  OutDataTypeStr=Inherit: Same as first input
  Product2 : Product  RequirementInfo={'doors' '00001143' '48' 'false' 'DOORS Surrogate Item' '' } %GIDa_0b375ef9_ec18_4b31_813b_9fb47ab25a89  Inputs=/*  SaturateOnIntegerOverflow=on  RndMeth=Zero  InputSameDT=on  OutDataTypeStr=Inherit: Same as first input
  "Sonic Flow " : Constant  RequirementInfo={'doors' '00001143' '49' 'false' 'DOORS Surrogate Item' '' } %GIDa_22b67916_0860_4f9d_9f6c_7dbd9ce931a3  Value=1.0
  Sum : Sum  RequirementInfo={'doors' '00001143' '50' 'false' 'DOORS Surrogate Item' '' } %GIDa_7707d992_0b7d_4c2a_92fa_136fb698da05  Inputs=+-  SaturateOnIntegerOverflow=on  InputSameDT=on  OutDataTypeStr=Inherit: Same as first input
  direction : Signum  RequirementInfo={'doors' '00001143' '51' 'false' 'DOORS Surrogate Item' '' } %GIDa_ace0228d_c2d0_4b06_aa6b_e0cc6315b334
  f(theta) : Fcn  RequirementInfo={'doors' '00001143' '52' 'false' 'DOORS Surrogate Item' '' } %GIDa_7ee0ff31_4a3a_4f07_916d_1b8b7866cc4f  Expr=2.821 - 0.05231*u[1] + 0.10299*u[1]*u[1] - 0.00063*u[1]*u[1]*u[1]
  g(pratio) : Fcn  RequirementInfo={'doors' '00001143' '53' 'false' 'DOORS Surrogate Item' '' } %GIDa_1eb9cf27_f7de_4919_ab5c_ed0def5f6969  Expr=2*sqrt(u - u*u)
  threshold = 0.5 : Switch  RequirementInfo={'doors' '00001143' '54' 'false' 'DOORS Surrogate Item' '' } %GIDa_a58493db_6d32_44cf_83fb_f9e9d5fdc402  Threshold=0.5  SaturateOnIntegerOverflow=on  InputSameDT=on
  "Throttle  Flow, mdot  (g/s)" : Outport  RequirementInfo={'doors' '00001143' '55' 'false' 'DOORS Surrogate Item' '' } %GIDa_a307216a_80c0_48c8_b7a9_581205d5216d  InitialOutput=0
  wires:
  "Manifold Pressure, Pm (bar)"/1 -> Sum/2, Product2/1, Product1/1
  Product2/1 -> MinMax/2
  Product1/1 -> MinMax/1
  "Atmospheric Pressure, Pa (bar) "/1 -> Sum/1, Product2/2, Product1/2
  g(pratio)/1 -> threshold = 0.5/1
  "Sonic Flow "/1 -> threshold = 0.5/3
  threshold = 0.5/1 -> Product/2
  direction/1 -> Product/3
  Sum/1 -> direction/1
  MinMax/1 -> threshold = 0.5/2, g(pratio)/1  "pratio"
  "Throttle Angle, theta (deg)"/1 -> f(theta)/1
  Product/1 -> "Throttle  Flow, mdot  (g/s)"/1
  f(theta)/1 -> Product/1

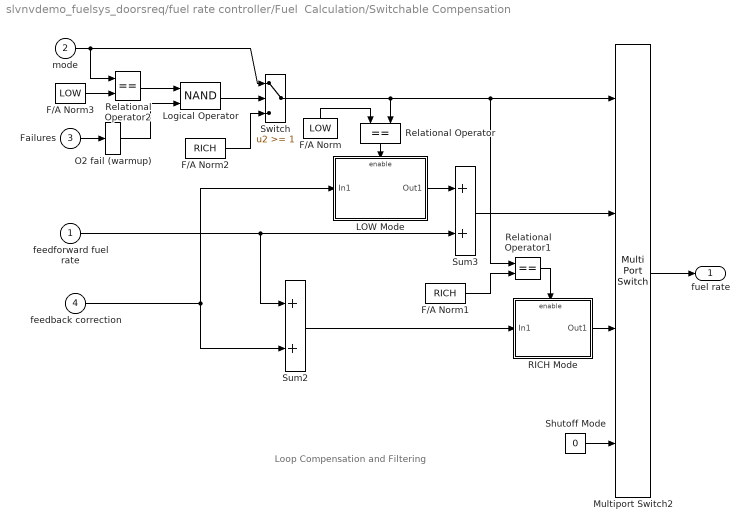
== system slvnvdemo_fuelsys_doorsreq/fuel rate controller/Fuel  Calculation/Switchable Compensation ==
  note: Loop Compensation and Filtering
  feedforward fuel rate : Inport  RequirementInfo={'doors' '00001143' '103' 'false' 'DOORS Surrogate Item' '' } %GIDa_61e65fa7_62f7_4f2e_8d0b_e259aeadd3c8
  mode : Inport  RequirementInfo={'doors' '00001143' '104' 'false' 'DOORS Surrogate Item' '' } %GIDa_58f7414e_02d7_44ba_9213_c6ec8d3c649a  Port=2
  Failures : Inport  RequirementInfo={'doors' '00001143' '105' 'false' 'DOORS Surrogate Item' '' } %GIDa_2753c7d2_7a5a_4c89_90c4_a5ca6db5a46d  Port=3
  feedback correction : Inport  RequirementInfo={'doors' '00001143' '106' 'false' 'DOORS Surrogate Item' '' } %GIDa_106a923e_3de8_46ee_839f_ca2a270c8646  Port=4
  F/A Norm : Constant  RequirementInfo={'doors' '00001143' '107' 'false' 'DOORS Surrogate Item' '' } %GIDa_cd3e7cdf_e36e_4979_85db_6eb2268233cb  Value=LOW
  F/A Norm1 : Constant  RequirementInfo={'doors' '00001143' '108' 'false' 'DOORS Surrogate Item' '' } %GIDa_ca84c86a_820b_4c29_8c18_94e821ee1db4  Value=RICH
  F/A Norm2 : Constant  RequirementInfo={'doors' '00001143' '109' 'false' 'DOORS Surrogate Item' '' } %GIDa_a8c2c872_d80c_4b85_8120_6ea6aa50deb2  Value=RICH
  F/A Norm3 : Constant  RequirementInfo={'doors' '00001143' '110' 'false' 'DOORS Surrogate Item' '' } %GIDa_a4d615e2_8806_4606_9cef_bec7185cb4b9  Value=LOW
  LOW Mode : Subsystem  RequirementInfo={'doors' '00001143' '111' 'false' 'DOORS Surrogate Item' '' } %GIDa_cbe299b8_e7c5_43fa_9756_12f46fdc6ed9  mask(enabled discrete-time transfer function){num=B1, den=A1, u0=-0.01, y0=-0.01, Ts=0.01}
      mask prompts: num "numerator polynomial"; den "denominator polynomial"; u0 "initial input"; y0 "initial output"; Ts "sample time"
      mask Display: dpoly(num,den,'z')
  Logical Operator : Logic  RequirementInfo={'doors' '00001143' '116' 'false' 'DOORS Surrogate Item' '' } %GIDa_70283f5c_6922_4ea6_b6f6_cda643039978  Operator=NAND
  Multiport Switch2 : MultiPortSwitch  RequirementInfo={'doors' '00001143' '117' 'false' 'DOORS Surrogate Item' '' } %GIDa_0d3a8565_5b5a_4e9a_a563_8a62be2ba420  zeroidx=off  SaturateOnIntegerOverflow=on  InputSameDT=on
  O2 fail (warmup) : Selector  RequirementInfo={'doors' '00001143' '118' 'false' 'DOORS Surrogate Item' '' } %GIDa_8235caf3_38bf_42be_b4c2_db4224345bfd  InputPortWidth=4  IndexOptions=Index vector (dialog)  Indices=3  OutputSizes=1
  RICH Mode : Subsystem  RequirementInfo={'doors' '00001143' '119' 'false' 'DOORS Surrogate Item' '' } %GIDa_753dbcca_3a7c_4f38_adf6_9bc2e05d25f4  mask(enabled discrete-time transfer function){num=B2, den=A2, u0=1.6, y0=1.6, Ts=0.01}
      mask prompts: num "numerator polynomial"; den "denominator polynomial"; u0 "initial input"; y0 "initial output"; Ts "sample time"
      mask Display: dpoly(num,den,'z')
  Relational Operator : RelationalOperator  RequirementInfo={'doors' '00001143' '124' 'false' 'DOORS Surrogate Item' '' } %GIDa_c4211654_bd22_49a3_ba1c_32715597df94  Operator===  InputSameDT=on
  Relational Operator1 : RelationalOperator  RequirementInfo={'doors' '00001143' '125' 'false' 'DOORS Surrogate Item' '' } %GIDa_7345f552_bea5_45bf_9145_561eee9e3ab9  Operator===  InputSameDT=on
  Relational Operator2 : RelationalOperator  RequirementInfo={'doors' '00001143' '126' 'false' 'DOORS Surrogate Item' '' } %GIDa_41d5e5d6_bdfe_41d7_bdb7_63f63f3f2550  Operator===  InputSameDT=on
  Shutoff Mode : Constant  RequirementInfo={'doors' '00001143' '127' 'false' 'DOORS Surrogate Item' '' } %GIDa_96259477_a876_4177_89b7_f47d19b7c758  Value=0
  Sum2 : Sum  RequirementInfo={'doors' '00001143' '128' 'false' 'DOORS Surrogate Item' '' } %GIDa_f00b5498_2220_44e1_be47_0a9b19352c4e  SaturateOnIntegerOverflow=on  InputSameDT=on  OutDataTypeStr=Inherit: Same as first input
  Sum3 : Sum  RequirementInfo={'doors' '00001143' '129' 'false' 'DOORS Surrogate Item' '' } %GIDa_718ea3d3_0505_4233_92f0_184d210ec9f8  SaturateOnIntegerOverflow=on  InputSameDT=on  OutDataTypeStr=Inherit: Same as first input
  Switch : Switch  RequirementInfo={'doors' '00001143' '130' 'false' 'DOORS Surrogate Item' '' } %GIDa_1f407643_f9c8_41e2_83d8_b5066e49b833  Threshold=1  SaturateOnIntegerOverflow=on  InputSameDT=on
  fuel rate : Outport  RequirementInfo={'doors' '00001143' '131' 'false' 'DOORS Surrogate Item' '' } %GIDa_98e8e5c9_a1ee_451e_a3f3_b70fc5e03e73  InitialOutput=0
  wires:
  feedforward fuel rate/1 -> Sum3/2, Sum2/1
  feedback correction/1 -> LOW Mode/1(In1), Sum2/2
  RICH Mode/1(Out1) -> Multiport Switch2/3
  LOW Mode/1(Out1) -> Sum3/1
  Sum3/1 -> Multiport Switch2/2
  Sum2/1 -> RICH Mode/1(In1)
  Shutoff Mode/1 -> Multiport Switch2/4
  F/A Norm1/1 -> Relational Operator1/2
  Relational Operator1/1 -> RICH Mode/Enable
  Relational Operator/1 -> LOW Mode/Enable
  Multiport Switch2/1 -> fuel rate/1
  Switch/1 -> Relational Operator1/1, Multiport Switch2/1, Relational Operator/2
  F/A Norm/1 -> Relational Operator/1
  F/A Norm2/1 -> Switch/3
  Logical Operator/1 -> Switch/2
  mode/1 -> Switch/1, Relational Operator2/1
  F/A Norm3/1 -> Relational Operator2/2
  Relational Operator2/1 -> Logical Operator/1
  Failures/1 -> O2 fail (warmup)/1
  O2 fail (warmup)/1 -> Logical Operator/2

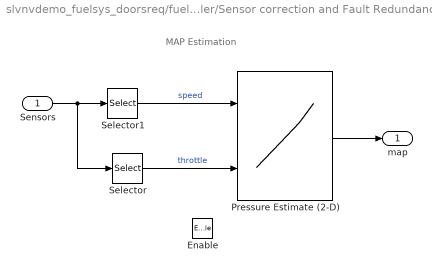
== system slvnvdemo_fuelsys_doorsreq/fuel rate controller/Sensor correction and Fault Redundancy/MAP Estimate ==
  note: MAP Estimation
  Sensors : Inport  RequirementInfo={'doors' '00001143' '141' 'false' 'DOORS Surrogate Item' '' } %GIDa_05175c58_1bec_465b_b75e_562238a0dc3f
  Enable : EnablePort  RequirementInfo={'doors' '00001143' '142' 'false' 'DOORS Surrogate Item' '' } %GIDa_7db9bdfa_24c0_42dd_b6f4_86d53f6a188e  PropagateVarSize=During execution
  Pressure Estimate (2-D) : Lookup2D  RequirementInfo={'doors' '00001143' '143' 'false' 'DOORS Surrogate Item' '' } %GIDa_64dea128_242f_4bef_878d_dfec22842d81  RowIndex=SpeedVect  ColumnIndex=ThrotVect  Table=PressEst  SaturateOnIntegerOverflow=on  InputSameDT=on
  Selector : Selector  RequirementInfo={'doors' '00001143' '144' 'false' 'DOORS Surrogate Item' '' } %GIDa_1ce53411_ec67_4c89_bb4e_da2a90b8b775  InputPortWidth=4  IndexOptions=Index vector (dialog)  Indices=1  OutputSizes=1
  Selector1 : Selector  RequirementInfo={'doors' '00001143' '145' 'false' 'DOORS Surrogate Item' '' } %GIDa_3c690e52_5d02_436b_8434_f75578f632b4  InputPortWidth=4  IndexOptions=Index vector (dialog)  Indices=2  OutputSizes=1
  map : Outport  RequirementInfo={'doors' '00001143' '146' 'false' 'DOORS Surrogate Item' '' } %GIDa_d0155bc3_e90e_4122_a334_a9a352ace6c4  InitialOutput=0
  wires:
  Sensors/1 -> Selector1/1, Selector/1
  Selector1/1 -> Pressure Estimate (2-D)/1  "speed"
  Selector/1 -> Pressure Estimate (2-D)/2  "throttle"
  Pressure Estimate (2-D)/1 -> map/1

== system slvnvdemo_fuelsys_doorsreq/fuel rate controller/Sensor correction and Fault Redundancy/Speed Estimate ==
  Sensors : Inport  RequirementInfo={'doors' '00001143' '149' 'false' 'DOORS Surrogate Item' '' } %GIDa_4c7e3ffa_1aa5_43ef_8399_d58014ef5a56
  Enable : EnablePort  RequirementInfo={'doors' '00001143' '150' 'false' 'DOORS Surrogate Item' '' } %GIDa_c92aba3b_6222_4917_8062_4095bcbbc690  PropagateVarSize=During execution
  Selector : Selector  RequirementInfo={'doors' '00001143' '151' 'false' 'DOORS Surrogate Item' '' } %GIDa_c2ae7328_dbd4_430b_a548_763b46c9775c  InputPortWidth=4  IndexOptions=Index vector (dialog)  Indices=1  OutputSizes=1
  Selector1 : Selector  RequirementInfo={'doors' '00001143' '152' 'false' 'DOORS Surrogate Item' '' } %GIDa_3d4ad04b_93ad_4bc6_b28b_503fcbb665f5  InputPortWidth=4  IndexOptions=Index vector (dialog)  Indices=4  OutputSizes=1
  Speed Table (2-D) : Lookup2D  RequirementInfo={'doors' '00001143' '153' 'false' 'DOORS Surrogate Item' '' } %GIDa_66690cc9_e023_4a7f_a9cc_49b2f123bb4e  RowIndex=ThrotVect  ColumnIndex=press  Table=SpeedEst  SaturateOnIntegerOverflow=on  InputSameDT=on
  we : Outport  RequirementInfo={'doors' '00001143' '154' 'false' 'DOORS Surrogate Item' '' } %GIDa_3935fb49_8375_419c_80b5_f4ce4f6d6cf2  InitialOutput=0
  wires:
  Speed Table (2-D)/1 -> we/1
  Sensors/1 -> Selector1/1, Selector/1
  Selector/1 -> Speed Table (2-D)/1  "throttle"
  Selector1/1 -> Speed Table (2-D)/2  "Manifold pressure"

== system slvnvdemo_fuelsys_doorsreq/fuel rate controller/Sensor correction and Fault Redundancy/Throttle Estimate ==
  Sensors : Inport  RequirementInfo={'doors' '00001143' '160' 'false' 'DOORS Surrogate Item' '' } %GIDa_3db58f68_6248_4007_ada5_7c8d313d5100
  Enable : EnablePort  RequirementInfo={'doors' '00001143' '161' 'false' 'DOORS Surrogate Item' '' } %GIDa_71929c39_8d37_443d_aac9_ab3f67de7039  PropagateVarSize=During execution
  Selector1 : Selector  RequirementInfo={'doors' '00001143' '162' 'false' 'DOORS Surrogate Item' '' } %GIDa_ef1e7f7b_df5e_45fb_b5c0_eacdeb0e0860  InputPortWidth=4  IndexOptions=Index vector (dialog)  Indices=4  OutputSizes=1
  Selector2 : Selector  RequirementInfo={'doors' '00001143' '163' 'false' 'DOORS Surrogate Item' '' } %GIDa_d8a5a767_2f16_45b2_990f_5157499e6dc3  InputPortWidth=4  IndexOptions=Index vector (dialog)  Indices=2  OutputSizes=1
  Thrott Estimation Table (2-D) : Lookup2D  RequirementInfo={'doors' '00001143' '164' 'false' 'DOORS Surrogate Item' '' } %GIDa_55d6afce_c1ae_4412_bf01_59bb9e179644  RowIndex=SpeedVect  ColumnIndex=press  Table=ThrotEst  SaturateOnIntegerOverflow=on  InputSameDT=on
  throttle : Outport  RequirementInfo={'doors' '00001143' '165' 'false' 'DOORS Surrogate Item' '' } %GIDa_87648f43_1a96_46b4_acec_628a90297b07  InitialOutput=0
  wires:
  Sensors/1 -> Selector2/1, Selector1/1
  Selector2/1 -> Thrott Estimation Table (2-D)/1  "speed"
  Selector1/1 -> Thrott Estimation Table (2-D)/2  "Manifold pressure"
  Thrott Estimation Table (2-D)/1 -> throttle/1

== system slvnvdemo_fuelsys_doorsreq/fuel rate controller/Fuel  Calculation/Switchable Compensation/LOW Mode ==
  In1 : Inport  RequirementInfo={'doors' '00001143' '112' 'false' 'DOORS Surrogate Item' '' } %GIDa_ab589b03_785a_4f3e_94f9_37acc6c8975f
  Enable : EnablePort  RequirementInfo={'doors' '00001143' '113' 'false' 'DOORS Surrogate Item' '' } %GIDa_395071aa_93de_4b01_b2f6_e9fd1dbcc693  StatesWhenEnabling=reset  PropagateVarSize=During execution
  Discrete Transfer Fcn (with initial outputs) : simulink_extras/Additional Discrete/Discrete Transfer Fcn (with initial outputs)  RequirementInfo={'doors' '00001143' '114' 'false' 'DOORS Surrogate Item' '' } %GIDa_6b834f97_7797_470d_be12_19ba2b6a32b8  SystemSampleTime=-1  N=num  D=den  U0=u0  Y0=y0  TS=Ts
  Out1 : Outport  RequirementInfo={'doors' '00001143' '115' 'false' 'DOORS Surrogate Item' '' } %GIDa_a478039d_c7d9_49bb_bea4_b14dbff0e67b  InitialOutput=y0
  wires:
  Discrete Transfer Fcn (with initial outputs)/1 -> Out1/1
  In1/1 -> Discrete Transfer Fcn (with initial outputs)/1

== system slvnvdemo_fuelsys_doorsreq/fuel rate controller/Fuel  Calculation/Switchable Compensation/RICH Mode ==
  In1 : Inport  RequirementInfo={'doors' '00001143' '120' 'false' 'DOORS Surrogate Item' '' } %GIDa_fe6598ed_81f3_4625_91f2_7570ec07422e
  Enable : EnablePort  RequirementInfo={'doors' '00001143' '121' 'false' 'DOORS Surrogate Item' '' } %GIDa_f07f6524_f62c_461f_86fb_12c2040d1fae  StatesWhenEnabling=reset  PropagateVarSize=During execution
  Discrete Transfer Fcn (with initial outputs) : simulink_extras/Additional Discrete/Discrete Transfer Fcn (with initial outputs)  RequirementInfo={'doors' '00001143' '122' 'false' 'DOORS Surrogate Item' '' } %GIDa_ea3b5061_2473_45ff_aba7_978de1831df3  SystemSampleTime=-1  N=num  D=den  U0=u0  Y0=y0  TS=Ts
  Out1 : Outport  RequirementInfo={'doors' '00001143' '123' 'false' 'DOORS Surrogate Item' '' } %GIDa_e928d8da_a0ec_49fa_9382_458fea2910d2  InitialOutput=y0
  wires:
  In1/1 -> Discrete Transfer Fcn (with initial outputs)/1
  Discrete Transfer Fcn (with initial outputs)/1 -> Out1/1

== stateflow chart fuel rate controller/control logic ==
  settings: updateMethod=DISCRETE  sampleTime=0.01
  state O2 [parallel]
    settings: executionOrder=1  description=This state determines the validity of the exhaust gas oxygen sensor (EGO) data.
    state fail
      entry: fail_state[O2] = 1;
      settings: description=The EGO sensor has failed.
    state warmup
      entry: fail_state[O2] = 1;
      settings: description=The EGO sensor must come up to temperature before its data is reliable.
    state normal
      entry: fail_state[O2] = 0;
      settings: description=Normal EGO sensor operation gives a reliable indication of excess oxygen in the exhaust gas, from which air/fuel mixture can be inferred.
    O2.fail -> O2.normal : [Ego < max_ego] /
        | Fail.DEC
    O2.normal -> O2.fail : [Ego > max_ego]/
        | Fail.INC
      settings: description=The failure condition is indicated by excessive output voltage.
    (default) -> warmup
    warmup -> O2.normal : [t > o2_t_thresh]
      settings: description=It is assumed that the time o2_t_thresh is sufficient for the sensor to warm up to operational temperature.
  state Pressure [parallel]
    settings: executionOrder=2  description=This state assesses the validity of the manifold absolute pressure (MAP) sensor.
    state normal
      entry:  fail_state[PRESS] = 0
      settings: description=The manifold pressure sensor gives a reliable indication of absolute pressure (MAP).
    state fail
      entry: fail_state[PRESS] = 1
      settings: description=The pressure sensor (manifold, or MAP) no longer produces reliable data.
    Pressure.normal -> Pressure.fail : [press > max_press | press < min_press]
        | /Fail.INC
    (default) -> Pressure.normal
    Pressure.fail -> Pressure.normal : [press > min_press & press < max_press] /
        | Fail.DEC
  state Throttle [parallel]
    settings: executionOrder=3  description=This state determines the validity of the throttle sensor signal.
    state normal
      entry: fail_state[THROT] = 0;
      settings: description=The throttle sensor gives a reliable indication of the angle of the throttle plate.
    state fail
      entry: fail_state[THROT] = 1;
      settings: description=Signal levels indicate that the throttle sensor data is no longer valid.
    Throttle.normal -> Throttle.fail : [throt> max_throt | throt < min_throt]/
        | Fail.INC
      settings: description=A failure is indicated by data which is outside the expected range, typically due to an open or short circuit.
    (default) -> Throttle.normal
    Throttle.fail -> Throttle.normal : [throt >  min_throt & throt < max_throt]
        | / Fail.DEC
  state Speed [parallel]
    settings: executionOrder=4  description="This state infers the validity of the speed sensor data.  A failure is indicated by the presence of manifold vacuum at zero speed."
    state normal
      entry: fail_state[SPEED] = 0
      settings: description=The speed sensor data accurately represents the engine speed.
    state fail
      entry: fail_state[SPEED] = 1
      settings: description=The engine speed data is no longer available.
    Speed.normal -> Speed.fail : [speed==0 & press < zero_thresh]/
        | Fail.INC
      settings: description="Loss of a reliable speed sensor signal will indicate zero speed.  This is deemed invalid when the manifold vacuum indicates otherwise."
    (default) -> Speed.normal
    Speed.fail -> Speed.normal : [speed > 0] /
        | Fail.DEC
  state Fail [parallel]
    settings: executionOrder=5  description=This state maintains a count of the number of sensors in failure mode.
    state Multi
      settings: description=This state represents any of the conditions in which more than one sensor is in failure mode.
      state Three
        settings: description=Three of the engine sensors have failed.
      state Four
        settings: description=All four of the engine sensors have failed.
      state Two
        settings: description=Two of the engine sensors have failed.
      Three -> Four [order 1] : INC
      Two -> Three [order 2] : INC
      Four -> Three : DEC
      Three -> Two [order 2] : DEC
    state One
      settings: description=One of the engine sensors has failed.
    state None
      settings: description=Zero failures; all sensors are operational.
    (default) -> None
    None -> One : INC
    One -> Two [order 1] : INC
    Two -> One [order 1] : DEC
    One -> None [order 2] : DEC
  state Fueling_Mode [parallel]
    settings: executionOrder=6  description=This state interprets the other states in the chart to directly control the fueling mode.
    state Fuel_Disabled
      entry: fuel_mode = DISABLED
      settings: description=The fuel is completely shut off while in this state.
      state Overspeed
        settings: description=The speed is dangerously high, so shut off the fuel.
      state Shutdown
        settings: description=Cut off system operation due to multiple sensor failures.
      Overspeed -> (junction 35) : [in(Speed.normal) & ...
          | speed < (max_speed - hys)]
      (junction 35) -> Shutdown [order 2] : [in(Fail.Multi)]
    state Running
      settings: description=The fuel is actively controlled while in this state.
      (history)
      state Low_Emissions
        entry: fuel_mode = LOW
        (history)
        state Normal
          settings: description=All sensors are in correct operating modes, so effective closed-loop mixture control can be used.
        state Warmup
          settings: description="The sensors are all operational, but the oxygen (EGO) sensor is warming up.  We'll target a stoichiometric ratio, nonetheless, but won't close the loop around exhaust gas oxygen."
        (junction 36) -> Normal [order 2]
        Warmup -> (junction 36) : [in(O2.normal)]
      state Rich_Mixture
        entry: fuel_mode = RICH
        settings: description=This mode enriches the mixture, lowering the air/fuel ratio.
        state Single_Failure
          settings: description=Continue uninterrupted engine operation, but with a richer mixture.
      Normal -> Single_Failure : [in(Fail.One)]
      Single_Failure -> Normal : [in(Fail.None)]
      (junction 36) -> Single_Failure [order 1] : [in(Fail.One)]
    Running -> Overspeed [order 2] : [ speed > max_speed ]
    (junction 35) -> Running [order 1] : [!in(Fail.Multi)]
    Running -> Shutdown [order 1] : enter(Fail.Multi)
    Shutdown -> Rich_Mixture : exit(Fail.Multi)
    (default) -> Warmup
  data: throt input double [0..120]; speed input double [0..1000]; Ego input double [0..12]; press input double [0..2]; fail_state output boolean size=4 [0..1]; fuel_mode output uint8 [1..3] =1; o2_t_thresh parameter double [0..60]; max_ego parameter double [0..2]; max_press parameter double [0..2]; min_press parameter double [0..2]; min_throt parameter double [0..120]; max_throt parameter double [0..120]; zero_thresh parameter double [0..450]; max_speed parameter double [0..1000]; hys parameter double [0..1000]; LOW parameter double; RICH parameter double; DISABLED parameter double; O2 constant uint8 =3; PRESS constant uint8 =4; THROT constant uint8 =1; SPEED constant uint8 =2
  data throt settings: description=throttle plate angle
  data speed settings: description=engine angular velocity
  data Ego settings: description=Exhaust Gas Oxygen
  data press settings: description=Manifold Absolute Pressure (MAP)
  data fail_state settings: description=array of failure indications for use by Simulink model
  data fuel_mode settings: description=fuel control mode: LOW = stoichiometric mixture, RICH = rich mixture, DISABLED = shut down
  data o2_t_thresh settings: description=Time required to warm the EGO sensor sufficiently for valid data.
  data max_ego settings: description=parameter represents the upper end of the EGO sensor range
  data max_press settings: description=parameter represents the upper limt of valid pressure readings
  data min_press settings: description=parameter for the lower end of the valid pressure sensor range
  data min_throt settings: description=minimum valid throttle angle
  data max_throt settings: description=parameter to indicate the maximum valid throttle angle reading
  data zero_thresh settings: description=minimum manifold pressure expected at zero speed
  data max_speed settings: description=parameter for the upper end of the safe engine speed range
  data hys settings: description=Hysteresis in the upper speed limit to avoid chatter at the threshold.
  data LOW settings: description="constant represents \"low emissions\" or stoichiometric fuel mixture mode"
  data RICH settings: description=constant represents rich fuel mixture mode
  data DISABLED settings: description=constant represents zero fuel mode
  data O2 settings: description=index into fail_state
  data PRESS settings: description=index into fail_state
  data THROT settings: description=index into fail_state
  events: DEC local EITHER_EDGE_EVENT; INC local EITHER_EDGE_EVENT
